simulink model "ammclib_mlib_rnd_s32k11x"  (Simulink 9.0)
settings: Solver=FixedStepDiscrete  StartTime=0.0  StopTime=5  FixedStep=0.001  RelTol=1e-3  EnableMultiTasking=on
InitFcn:
  | mbd_s32k_consistency_checks(bdroot(gcs));
undefined symbols (not defined in the file): LQFP, thumb
libraries: simulink x4, ammclib_bam_s32k11x x4, mbd_s32k1xx_ec_toolbox x2
Description:
  | This model tests the AMMCLIB MLIB RND blocks
  | 
  | Validation:
  | - Run the model in Simulation and compare the Inputs vs Outputs results.
  | - Open Freemaster (ammclib_mlib_rnd_s32k11x.pmp) and compare the HW results against the Simulated ones
  | 
  | E.g.: IF (RND_Input = 0.375) AND (u16In2 = 13) THEN output on ROUND_F16 should be 0x4000 ~ FRAC16(0.5)
  | E.g.: IF (RND_Input = 0.375) AND (u16In2 = 29) THEN output on ROUND_F32 should be FRAC32(0.5)
settings Model: Creator=NXP MBDT Team  LastModifiedBy=nxf35172
settings DataIOCC: ExternalInput=off  InitialState=off  LimitDataPoints=on  SaveOutput=off  SignalLogging=off  SaveTime=off
settings OptimizationCC: DefaultParameterBehavior=Inlined  PassReuseOutputArgsAs=Individual arguments  LifeSpan=auto
settings DebuggingCC: SolverPrmCheckMsg=warning  InheritedTsInSrcMsg=none  SingleTaskRateTransMsg=error  ParameterPrecisionLossMsg=none  ParameterTunabilityLossMsg=error  UnconnectedInputMsg=error  UnconnectedOutputMsg=error  UnconnectedLineMsg=error  AllowSymbolicDim=off  UnknownTsInhSupMsg=error  StateNameClashWarn=warning
settings HardwareCC: ProdLargestAtomicInteger=Long  ProdLargestAtomicFloat=Double  ProdIntDivRoundTo=Zero  ProdEndianess=LittleEndian  ProdHWDeviceType=ARM Compatible->ARM Cortex
settings SFSimCC: MATLABDynamicMemAlloc=off
settings RTWCC: SystemTargetFile=mbd_s32k.tlc  MakeCommand=mbd_s32k_make_rtw COPY_MDLREF_INCLUDES=0  TemplateMakefile=mbd_s32k.tmf  Description=Model Based Design Toolbox S32K14x Code Generation Target  GenerateReport=on  IncludeHyperlinkInReport=on  LaunchReport=on  GenerateTraceInfo=on  GenerateTraceReport=on  GenerateTraceReportSl=on  GenerateTraceReportSf=on  GenerateTraceReportEml=on
settings CodeAppCC: ForceParamTrailComments=on  IgnoreCustomStorageClasses=off  OperatorAnnotations=on  SimulinkDataObjDesc=on  SFDataObjDesc=on  InsertBlockDesc=on  StateflowObjectComments=off
settings STFCustomTargetCC: MultiwordLength=256  ModelReferenceCompliant=off  CombineOutputUpdateFcns=on  ERTCustomFileBanners=on  SupportContinuousTime=off  SupportNonInlinedSFcns=off  RemoveResetFunc=on  MATLABClassNameForMDSCustomization=Simulink.SoftwareTarget.ERTCustomization  GRTInterface=off  SystemTargetFile=mbd_s32k.tlc
settings ERTTargetCC: ModelReferenceCompliant=off  ParMdlRefBuildCompliant=off  CompOptLevelCompliant=off  ConcurrentExecutionCompliant=off  ModelStepFunctionPrototypeControlCompliant=off  CPPClassGenCompliant=off  UseToolchainInfoCompliant=off  InlinedParameterPlacement=NonHierarchical  ERTCustomFileTemplate=example_file_process.tlc

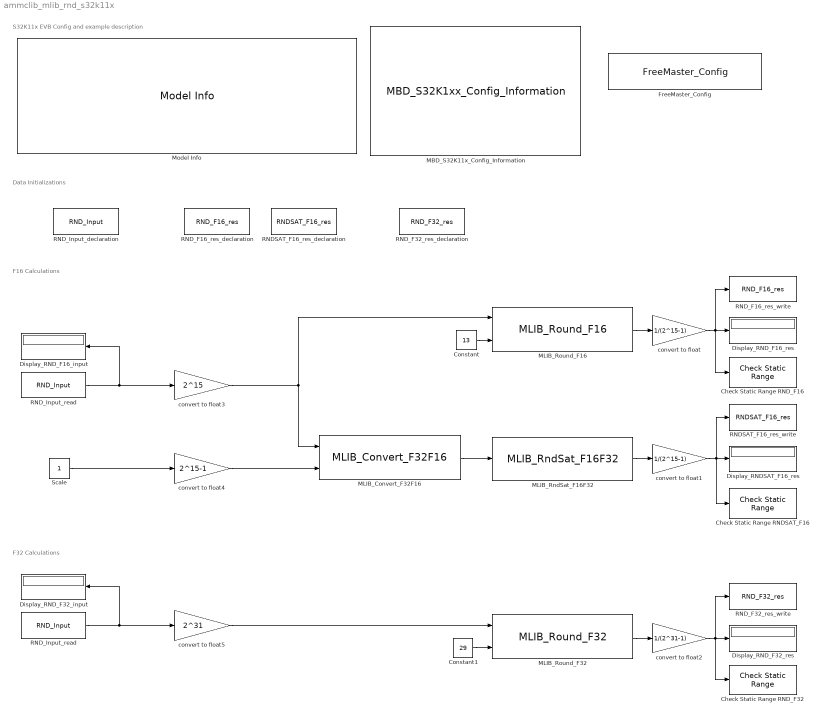
== system ammclib_mlib_rnd_s32k11x ==
  note: S32K11x EVB Config and example description
  note: Data Initializations
  note: F16 Calculations
  note: F32 Calculations
  "Check Static Range RNDSAT_F16 " : simulink/Model Verification/Check  Static Range  Description=0.36 <= u <= 0.38  max=0.38  max_included=on  min=0.36  min_included=on  enabled=on  stopWhenAssertionFail=on  export=off  icon=graphic
      settings: SourceProductName=Simulink  SourceProductBaseCode=SL
  Check Static Range RND_F16 : simulink/Model Verification/Check  Static Range  Description=0.4999 <= u <= 0.5001  max=0.5001  max_included=on  min=0.4999  min_included=on  enabled=on  stopWhenAssertionFail=on  export=off  icon=graphic
      settings: SourceProductName=Simulink  SourceProductBaseCode=SL
  Check Static Range RND_F32 : simulink/Model Verification/Check  Static Range  Description=0.4999 <= u <= 0.5001  max=0.5001  max_included=on  min=0.4999  min_included=on  enabled=on  stopWhenAssertionFail=on  export=off  icon=graphic
      settings: SourceProductName=Simulink  SourceProductBaseCode=SL
  Constant : Constant  Value=13  OutDataTypeStr=Inherit: Inherit via back propagation
  Constant1 : Constant  Value=29  OutDataTypeStr=Inherit: Inherit via back propagation
  Display_RNDSAT_F16_res : Display
  Display_RND_F16_input : Display
  Display_RND_F16_res : Display
  "Display_RND_F32_input " : Display
  Display_RND_F32_res : Display
  FreeMaster_Config : mbd_s32k1xx_ec_toolbox/Utility Blocks/FreeMaster_Config  interface=LPUART0  baudrate=19200  rxd=PTB0: [LPUART0_RX | Receive]  txd=PTB1: [LPUART0_TX | Transmit]  mode=Short Interrupt  isr_prio=3  show_adv_opts=on  use_scope=on  max_scope_vars=8  use_recorder=on  max_rec_vars=8  rec_buff_size=1024  rec_timebase=0 seconds  comm_buffer_size_auto=on  comm_buffer_size=255  comm_rqueue_size_default=on  comm_rqueue_size=32
  MBD_S32K11x_Config_Information : mbd_s32k1xx_ec_toolbox/MBD_S32K1xx_Config_Information  mbdt_ver=0  disp_str=|  config_params=[]  mcu_target_name=S32K116  mcu_target_package=48-LQFP  mcu_target_sram_size=17KB  mcu_system_clock_freq=40  mcu_xtal_freq=External 40  mcu_steptick_timer=LPIT Channel 0  mcu_steptick_prio=3  ds_import_enable=on  target_compiler=GCC  target_memory=FLASH  gcc_target_compile_opts=-mcpu=cortex-m0plus -mthumb -O1 -g -gstrict-dwarf  gcc_target_assemble_opts=-mcpu=cortex-m0plus -mthumb -g  gcc_target_link_opts=-mcpu=cortex-m0plus -mthumb  gcc_target_default_lcf=on  gcc_target_user_lcf=S32K116_17_flash.ld  ghs_target_compile_opts=-mcpu=cortexm0plus -mthumb -fsoft -Ogeneral -Wundef -Wimplicit-int -Wshadow -Wtrigraphs --no_commons --gnu_asm -gnu99 -gdwarf-2 -G  ghs_target_assemble_opts=-mcpu=cortexm0plus -mthumb -fsoft --gnu_asm  ghs_target_link_opts=-mcpu=cortexm0plus -mthumb -fsoft  ghs_target_default_lcf=on  ghs_target_user_lcf=S32K116_17_flash.ld  iar_target_compile_opts=--thumb -Ol -e --debug --dlib_config normal  iar_target_assemble_opts=--thumb  iar_target_link_opts=--no_exceptions --vfe --inline  iar_target_default_lcf=on  iar_target_user_lcf=S32K116_17_flash.icf  pil_download_enable=off  rbl_download_enable=on  rbl_start_delay=5000  rbl_download_interface=OpenSDA  rbl_restart_request=off  rbl_com_port=Custom  rbl_com_port_custom=COM1  pil_download_rate=57600  pil_opensda_drive=Custom  pil_opensda_drive_custom=D  pil_uart_instance=0  pil_uart_rx=PTB0: [LPUART0_RX | Receive]  pil_uart_tx=PTB1: [LPUART0_TX | Transmit]  FTM_PWM_PcrCheckEnDis=on  FTM_Input_Edge_Inputs_PcrCheckEnDis=on  FTM_Dual_Edge_Inputs_PcrCheckEnDis=on  FTM_Quadrature_Inputs_PcrCheckEnDis=on  FTM_Hall_Sensor_Inputs_PcrCheckEnDis=on  LPTMR_PcrCheckEnDis=on  PIT_PcrCheckEnDis=on  RTC_PcrCheckEnDis=on  FlexCAN_PcrCheckEnDis=on  LIN_PcrCheckEnDis=on  FlexIO_PcrCheckEnDis=on  LPI2C_PcrCheckEnDis=on  LPSPI_PcrCheckEnDis=on  LPUART_PcrCheckEnDis=on  CMP_PcrCheckEnDis=on  GPIO_OutputPcrCheckEnDis=on  GPIO_InputPcrCheckEnDis=on  SBC_PcrCheckEnDis=on  AMMCLIB_PcrCheckEnDis=on  FM_PcrCheckEnDis=on  Profile_PcrCheckEnDis=on  ConfigParams_PcrCheckEnDis=on  ModelRef_PcrCheckEnDis=on  PDB0_PcrCheckEnDis=on  CSEc_PcrCheckEnDis=on  eDMA_PcrCheckEnDis=on  ADC_PcrCheckEnDis=on  WDOG_PcrCheckEnDis=on
      | Target : S32K144-64KB_SRAM
      | Package : 100-pin
      | System clock : 80 MHz
      | XTAL clock : External 8 MHz
      | Compiler : IAR
      | Target Type : FLASH
      | Download Code after build : off
      | Step Tick Interrupt Priority : 15
  MLIB_Convert_F32F16 : ammclib_bam_s32k11x/MLIB/bam_f32/MLIB_Convert_F32F16
  MLIB_RndSat_F16F32 : ammclib_bam_s32k11x/MLIB/bam_f16/MLIB_RndSat_F16F32
  MLIB_Round_F16 : ammclib_bam_s32k11x/MLIB/bam_f16/MLIB_Round_F16
  MLIB_Round_F32 : ammclib_bam_s32k11x/MLIB/bam_f32/MLIB_Round_F32
  Model Info : simulink/Model-Wide Utilities/Model Info  Frame=off  DisplayStringWithTags=|  HorizontalTextAlignment=Left  LeftAlignmentValue=0.02
      | Model Name: %<ModelName>
      | 
      | Description: %<Description>
  RNDSAT_F16_res_declaration : DataStoreMemory  Priority=3  DataStoreName=RNDSAT_F16_res  ReadBeforeWriteMsg=warning  WriteAfterWriteMsg=warning  WriteAfterReadMsg=warning  ShowAdditionalParam=off  OutDataTypeStr=single
  RNDSAT_F16_res_write : DataStoreWrite  DataStoreName=RNDSAT_F16_res
  RND_F16_res_declaration : DataStoreMemory  Priority=2  DataStoreName=RND_F16_res  ReadBeforeWriteMsg=warning  WriteAfterWriteMsg=warning  WriteAfterReadMsg=warning  ShowAdditionalParam=off  OutDataTypeStr=single
  RND_F16_res_write : DataStoreWrite  DataStoreName=RND_F16_res
  RND_F32_res_declaration : DataStoreMemory  Priority=2  DataStoreName=RND_F32_res  ReadBeforeWriteMsg=warning  WriteAfterWriteMsg=warning  WriteAfterReadMsg=warning  ShowAdditionalParam=off  OutDataTypeStr=single
  RND_F32_res_write : DataStoreWrite  DataStoreName=RND_F32_res
  RND_Input_declaration : DataStoreMemory  Priority=1  DataStoreName=RND_Input  WriteAfterWriteMsg=warning  WriteAfterReadMsg=warning  InitialValue=0.375  ShowAdditionalParam=off  OutMin=-1  OutMax=1  OutDataTypeStr=single
  RND_Input_read : DataStoreRead  DataStoreName=RND_Input
  "RND_Input_read " : DataStoreRead  DataStoreName=RND_Input
  Scale : Constant  OutDataTypeStr=Inherit: Inherit via back propagation
  convert to float : Gain  Gain=1/(2^15-1)  OutDataTypeStr=Inherit: Inherit via back propagation
  convert to float1 : Gain  Gain=1/(2^15-1)  OutDataTypeStr=Inherit: Inherit via back propagation
  convert to float2 : Gain  Gain=1/(2^31-1)  OutDataTypeStr=Inherit: Inherit via back propagation
  convert to float3 : Gain  Gain=2^15  ParamDataTypeStr=double  OutDataTypeStr=int16
  convert to float4 : Gain  Gain=2^15-1  ParamDataTypeStr=double  OutDataTypeStr=int16
  convert to float5 : Gain  Gain=2^31  OutDataTypeStr=Inherit: Inherit via back propagation
  wires:
  RND_Input_read/1 -> convert to float3/1, Display_RND_F16_input/1
  convert to float3/1 -> MLIB_Convert_F32F16/1, MLIB_Round_F16/1
  convert to float/1 -> RND_F16_res_write/1, Display_RND_F16_res/1, Check Static Range RND_F16/1
  MLIB_Round_F16/1 -> convert to float/1
  MLIB_RndSat_F16F32/1 -> convert to float1/1
  convert to float1/1 -> Display_RNDSAT_F16_res/1, RNDSAT_F16_res_write/1, "Check Static Range RNDSAT_F16 "/1
  "RND_Input_read "/1 -> convert to float5/1, "Display_RND_F32_input "/1
  convert to float5/1 -> MLIB_Round_F32/1
  convert to float2/1 -> RND_F32_res_write/1, Display_RND_F32_res/1, Check Static Range RND_F32/1
  MLIB_Round_F32/1 -> convert to float2/1
  Constant/1 -> MLIB_Round_F16/2
  Scale/1 -> convert to float4/1
  MLIB_Convert_F32F16/1 -> MLIB_RndSat_F16F32/1
  convert to float4/1 -> MLIB_Convert_F32F16/2
  Constant1/1 -> MLIB_Round_F32/2
